simulink model "Straight_cs_old"  (R2016a)
settings: Solver=ode5  SolverMode=SingleTasking  StartTime=0.0  StopTime=30  FixedStep=1/1000  RelTol=1e-3
PreLoadFcn:
  | mbxruntime.callbacks.PreLoadFcn(bdroot);
PostLoadFcn:
  | mbxruntime.callbacks.PostLoadFcn(bdroot);
InitFcn:
  | mbxruntime.callbacks.InitFcn(bdroot);
StartFcn:
  | mbxruntime.callbacks.StartFcn(bdroot);
StopFcn:
  | mbxruntime.callbacks.StopFcn(bdroot);
model workspace (MAT data in the model file):
  mbox_table : struct (value not decoded)
  model_closed = 0
  sim_status = 0
values from neighbouring files (symbols this model uses):
  ACCDuration = 5    [PreScan_Runscript.m]
  V0 = ACCArray(2*ACCCasei-1)    [PreScan_Runscript.m]
  V1 = ACCArray(2*ACCCasei)    [PreScan_Runscript.m]
  VAccuracyIn = 0.8    [PreScan_Runscript.m]
  VDurationIn = 2    [PreScan_Runscript.m]
  VPIDIn = ACCArray(2*ACCCasei-1)    [PreScan_Runscript.m]
  VToleranceIn = 1    [PreScan_Runscript.m]
undefined symbols (not defined in the file or in its folder): ADASID, BMotor1, BMotor2, BrkDelayTime, DControlB, Delay1, Delay2, DiscIntNeverNeededParam, IControlB, JMotor1, JMotor2, mbxruntime, PControlB, PreScanCarSimLoadFcn, ratioGearF, ratioGearR, tabledata, TorqDelayTime, Tstep
undefined symbols (not defined in the file): SteeringColumn, SteeringWheel, WheelL0, WheelL1, WheelR0, WheelR1
libraries: simulink x14, simulink_extras x10, MyLib x3, PreScanSimulinkLibrary x3, Solver_SF x2, PreScanUsefulBlocks x2, pil_lib x1
(part 2 of 11)

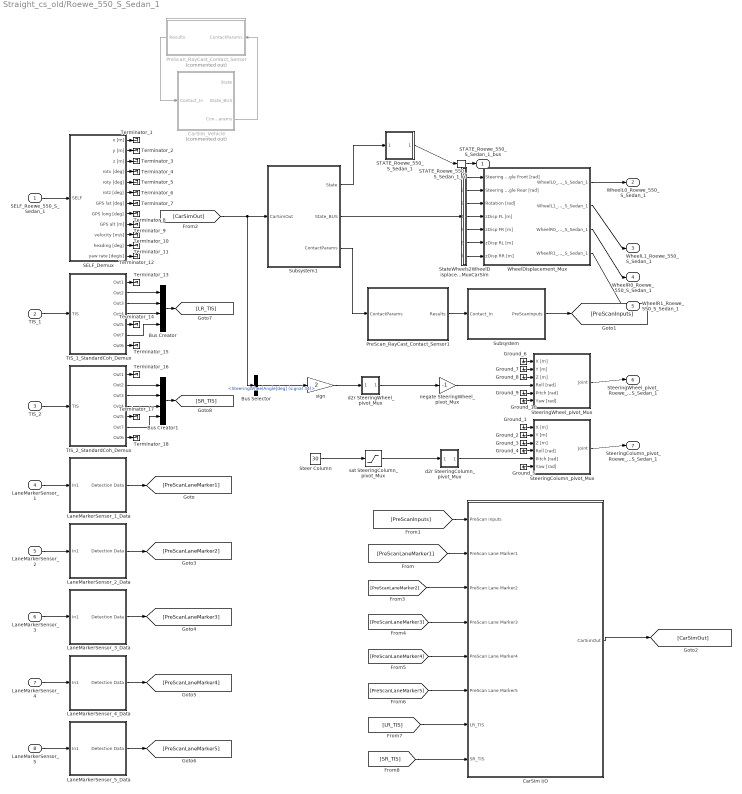
== system Straight_cs_old/Roewe_550_S_Sedan_1 ==
  SELF_Roewe_550_S_Sedan_1 : Inport  Tag=inport/SelfPort  OutDataTypeStr=Bus: PRESCAN_SELFSENSORDATA  PortDimensions=1  SampleTime=10/1000  BusOutputAsStruct=on
  TIS_1 : Inport  Tag=inport/TIS  Port=2  OutDataTypeStr=Bus: PRESCAN_SCANNERSENSOR_MESSAGE  PortDimensions=32  SampleTime=1/20  BusOutputAsStruct=on
  TIS_2 : Inport  Tag=inport/TIS  Port=3  OutDataTypeStr=Bus: PRESCAN_SCANNERSENSOR_MESSAGE  PortDimensions=32  SampleTime=1/20  BusOutputAsStruct=on
  LaneMarkerSensor_1 : Inport  Tag=inport/LaneMarker  Port=4  OutDataTypeStr=Bus: PRESCAN_LANEMARKER_MESSAGE  PortDimensions=4  SampleTime=1/20  BusOutputAsStruct=on
  LaneMarkerSensor_2 : Inport  Tag=inport/LaneMarker  Port=5  OutDataTypeStr=Bus: PRESCAN_LANEMARKER_MESSAGE  PortDimensions=4  SampleTime=1/20  BusOutputAsStruct=on
  LaneMarkerSensor_3 : Inport  Tag=inport/LaneMarker  Port=6  OutDataTypeStr=Bus: PRESCAN_LANEMARKER_MESSAGE  PortDimensions=4  SampleTime=1/20  BusOutputAsStruct=on
  LaneMarkerSensor_4 : Inport  Tag=inport/LaneMarker  Port=7  OutDataTypeStr=Bus: PRESCAN_LANEMARKER_MESSAGE  PortDimensions=4  SampleTime=1/20  BusOutputAsStruct=on
  LaneMarkerSensor_5 : Inport  Tag=inport/LaneMarker  Port=8  OutDataTypeStr=Bus: PRESCAN_LANEMARKER_MESSAGE  PortDimensions=4  SampleTime=1/20  BusOutputAsStruct=on
  Bus Creator : BusCreator  Inputs=4
  Bus Creator1 : BusCreator  Inputs=4
  Bus Selector : BusSelector  OutputSignals=SteeringWheelAngle[deg] (signal 34)
  CarSim I/O : Subsystem
  CarSim_Vehicle : Subsystem  Tag=UserSpecified_Subsys  Description=..\..\..\Program Files (x86)\CarSim201601_Data\Extensions\Simulink\CarSim_VehicleDynamics.mdl  Commented=on  LoadFcn=PreScanCarSimLoadFcn();  mask(User specified subsystem){update=off, sourcefilename=..\..\..\Program Files (x86)\CarSim201601_Data\Extensions\Simulink\CarSim_VehicleDynamics.mdl}
      mask prompts: update "Update (default: not checked)"; sourcefilename "Source file name"
      mask help:
      | A User-specified model may be selected as Controller or Dynamics of the vehicle. PreScan will copy the contents of the User-specified model into the user-specified model block.
      |
      | If update checkbox is checked the current user-specified model block will be deleted and will be REPLACED by (new) user specified model blocks. So, the current user specified model elements will be lost.
      |
      | Warning: If a new user-specified model is selected in the GUI, the user-specified model will be replaced.
      settings: DeleteFcn=PreScanBlockDeleteFcn;
      mask Help: eval('openHelp(227)')
      mask Display: userSpecifiedDynamics_mask_display();
  Ground_{1..10} (10 alike) : Ground
  LaneMarkerSensor_1_Data : Subsystem  Tag=demux/LaneMarkerSensor  mask{NUMBEROFSLICES=4, TimeStep=1/20}
      mask prompts: NUMBEROFSLICES "Number of slices"; TimeStep "Auto Assigned: Time Step [s]"
      mask Help: eval('openHelp(2301)')
  LaneMarkerSensor_2_Data : Subsystem  Tag=demux/LaneMarkerSensor  mask{NUMBEROFSLICES=4, TimeStep=1/20}
      mask prompts: NUMBEROFSLICES "Number of slices"; TimeStep "Auto Assigned: Time Step [s]"
      mask Help: eval('openHelp(2301)')
  LaneMarkerSensor_3_Data : Subsystem  Tag=demux/LaneMarkerSensor  mask{NUMBEROFSLICES=4, TimeStep=1/20}
      mask prompts: NUMBEROFSLICES "Number of slices"; TimeStep "Auto Assigned: Time Step [s]"
      mask Help: eval('openHelp(2301)')
  LaneMarkerSensor_4_Data : Subsystem  Tag=demux/LaneMarkerSensor  mask{NUMBEROFSLICES=4, TimeStep=1/20}
      mask prompts: NUMBEROFSLICES "Number of slices"; TimeStep "Auto Assigned: Time Step [s]"
      mask Help: eval('openHelp(2301)')
  LaneMarkerSensor_5_Data : Subsystem  Tag=demux/LaneMarkerSensor  mask{NUMBEROFSLICES=4, TimeStep=1/20}
      mask prompts: NUMBEROFSLICES "Number of slices"; TimeStep "Auto Assigned: Time Step [s]"
      mask Help: eval('openHelp(2301)')
  PreScan_RayCast_Contact_Sensor : Subsystem  Tag=PreScan_RayCast_Contact_Sensor  Commented=on  LoadFcn=|  mask(PreScan Block: PreScan RayCast Contact Sensor){x0=-95.5472, y0=-0.064154, z0=0, Roll0=0, Pitch0=0, Yaw0=0, wheelRadius=0.44999998807907104, hcog=0, b=2.7049999237060547, TimeStep=-1}
      | load PrescanXYZData;
      | load PrescanRPYData;
      | load PrescanQuatData;
      | load PrescanAxisAngleData;
      | load PrescanPoseData;
      | load PrescanPoseQData;
      | load PrescanPoseAData;
      | load PrescanWheelContactData;
      mask prompts: x0 "Ini x-position VEHICLE wrt GLOBAL axis system [m]"; y0 "Ini y-position VEHICLE wrt GLOBAL axis system [m]"; z0 "Ini z-position VEHICLE wrt GLOBAL axis system [m]"; Roll0 "Ini roll-angle BODY wrt VEHICLE axis system [deg]"; Pitch0 "Ini pitch-angle BODY wrt VEHICLE axis system [deg]"; Yaw0 "Ini yaw-angle VEHICLE wrt GLOBAL axis system [deg]"; wheelRadius "Wheel Radius [m]"; hcog "Dynamics: hCoG [m]"; b "Dynamics: b [m]"; TimeStep "Time Step [s]"
      mask help:
      | This block encapsulates the base Contact sensor.
      |
      | It takes input parameters from the PreScan 3D vehicle dynamics block and outputs contact results.
      mask Help: eval('openHelp(251)')
  PreScan_RayCast_Contact_Sensor1 : Subsystem  Tag=PreScan_RayCast_Contact_Sensor  LoadFcn=|  mask(PreScan Block: PreScan RayCast Contact Sensor){x0=-2.6473, y0=0.062788, z0=0, Roll0=0, Pitch0=0, Yaw0=0, wheelRadius=0.44999998807907104, hcog=0, b=2.7049999237060547, TimeStep=-1}
      | load PrescanXYZData;
      | load PrescanRPYData;
      | load PrescanQuatData;
      | load PrescanAxisAngleData;
      | load PrescanPoseData;
      | load PrescanPoseQData;
      | load PrescanPoseAData;
      | load PrescanWheelContactData;
      mask prompts: x0 "Ini x-position VEHICLE wrt GLOBAL axis system [m]"; y0 "Ini y-position VEHICLE wrt GLOBAL axis system [m]"; z0 "Ini z-position VEHICLE wrt GLOBAL axis system [m]"; Roll0 "Ini roll-angle BODY wrt VEHICLE axis system [deg]"; Pitch0 "Ini pitch-angle BODY wrt VEHICLE axis system [deg]"; Yaw0 "Ini yaw-angle VEHICLE wrt GLOBAL axis system [deg]"; wheelRadius "Wheel Radius [m]"; hcog "Dynamics: hCoG [m]"; b "Dynamics: b [m]"; TimeStep "Time Step [s]"
      mask help:
      | This block encapsulates the base Contact sensor.
      |
      | It takes input parameters from the PreScan 3D vehicle dynamics block and outputs contact results.
      mask Help: eval('openHelp(251)')
  SELF_Demux : Subsystem  Tag=demux/SelfPort  mask(PreScan Demux Block:){}
      mask help:
      | The SELF port shows (state) information of the actor itself. The outputs are position in the experiment's axis system and the GPS coordinates, and the object's absolute velocity and compass heading.
      |
      | For more information, please click Help.
      settings: DeleteFcn=PreScanBlockDeleteFcn;
      mask Help: eval('openHelp(462)')
      mask Display:
      | port_label('output',1,'x [m]')
      | port_label('output',2,'y [m]')
      | port_label('output',3,'z [m]','texmode','on')
      | port_label('output',4,'Rotx [deg]','texmode','on')
      | port_label('output',5,'Roty [deg]','texmode','on')
      | port_label('output',6,'Rotz [deg]','texmode','on')
      | port_label('output',7,'GPS lat [deg]','texmode','on')
      | port_label('output',8,'GPS long [deg]','texmode','on')
      | port_label('output',9,'GPS alt [m]','texmode','on')
      | port_label('output',10,'Velocity [m/s]')
      | port_label('output',11,'Heading [deg]')
      | port_label('output',12,'Yaw rate [deg/s]')
  STATE_Roewe_550_S_Sedan_1 : Subsystem  Tag=mux/StatePort  Priority=0  LoadFcn=load PrescanStateActuatorData  mask(PreScan Sink Block: State){x0=-95.5472, y0=-0.064154, z0=0, Roll0=0, Pitch0=0, Yaw0=0, TimeStep=1/1000}
      mask prompts: x0 "Ini x-position VEHICLE wrt GLOBAL axis system [m]"; y0 "Ini y-position VEHICLE wrt GLOBAL axis system [m]"; z0 "Ini z-position VEHICLE wrt GLOBAL axis system [m]"; Roll0 "Ini roll-angle BODY wrt VEHICLE axis system [deg]"; Pitch0 "Ini pitch-angle BODY wrt VEHICLE axis system [deg]"; Yaw0 "Ini yaw-angle VEHICLE wrt GLOBAL axis system [deg]"; TimeStep "Auto-Assigned: Upload Period [s]"
      mask help:
      | The Actor State contains a vector signal of size (9x1), containing the following signals:
      |
      | -  Position                  (x,y,z)                                     [m]
      | -  Velocity                  (vx,vy,vz)                               [m/s]
      | -  Angles                    (Roll, Pitch, Yaw)                   [rad]
      |
      | The Actor state is defined in the global axis system.
      | The state is superponed on the Initial position defined in the GUI.
      |
      | For more information, please click Help.
      settings: DeleteFcn=PreScanBlockDeleteFcn;
      mask Help: eval('openHelp(222)')
      mask Display: image(imread('State.png'))
  STATE_Roewe_550_S_Sedan_1_rc : RateTransition  Tag=mux_rc/StatePort  OutPortSampleTimeOpt=Inherit
  StateWheels2WheelDisplacementMuxCarSim : Subsystem  Tag=StateWheels2WheelDisplacementMuxCarSim  mask(PreScan Utility Block:){}
      mask help: This block selects the CarSim wheels displacement and rotation.
      settings: DeleteFcn=PreScanBlockDeleteFcn;
  Steer Column : Constant  Value=30
  SteeringColumn_pivot_Mux : Subsystem  Tag=mux/Joint  mask(PreScan Mux Block){DisplayName=SteeringColumn}
      mask prompts: DisplayName "Display Name"
      mask help:
      | This block simulates a generic joint used for generic models. This joint can be enabled/disabled from the GUI.
      |
      | For more information, please click Help.
      settings: DeleteFcn=PreScanBlockDeleteFcn;
      mask Help: eval('openHelp(254)')
  SteeringWheel_pivot_Mux : Subsystem  Tag=mux/Joint  mask(PreScan Mux Block){DisplayName=SteeringWheel}
      mask prompts: DisplayName "Display Name"
      mask help:
      | This block simulates a generic joint used for generic models. This joint can be enabled/disabled from the GUI.
      |
      | For more information, please click Help.
      settings: DeleteFcn=PreScanBlockDeleteFcn;
      mask Help: eval('openHelp(254)')
  Subsystem : Subsystem
  Subsystem1 : Subsystem
  TIS_1_StandardCoh_Demux : Subsystem  Tag=demux/TIS/StandardCoh  TreatAsAtomicUnit=on  mask(PreScan Demux Block: TIS){MAXMESSAGES=32}
      mask prompts: MAXMESSAGES "Number of Objects"
      mask Help: eval('openHelp(449)')
      mask Display:
      | port_label('input',1,'TIS')
      | port_label('output',1,'Beam ID [-]')
      | port_label('output',2,'Range [m]')
      | port_label('output',3,'DopplerVelocity [m/s]')
      | port_label('output',4,'{\theta} [deg]','texmode','on')
      | port_label('output',5,'{\phi} [deg]','texmode','on')
      | port_label('output',6,'Target ID [-]','texmode','on')
      | port_label('output',7,'TIS Data','texmode','on')
  TIS_2_StandardCoh_Demux : Subsystem  Tag=demux/TIS/StandardCoh  TreatAsAtomicUnit=on  mask(PreScan Demux Block: TIS){MAXMESSAGES=32}
      mask prompts: MAXMESSAGES "Number of Objects"
      mask Help: eval('openHelp(449)')
      mask Display:
      | port_label('input',1,'TIS')
      | port_label('output',1,'Beam ID [-]')
      | port_label('output',2,'Range [m]')
      | port_label('output',3,'DopplerVelocity [m/s]')
      | port_label('output',4,'{\theta} [deg]','texmode','on')
      | port_label('output',5,'{\phi} [deg]','texmode','on')
      | port_label('output',6,'Target ID [-]','texmode','on')
      | port_label('output',7,'TIS Data','texmode','on')
  Terminator_{1..18} (18 alike) : Terminator
  WheelDisplacement_Mux : Subsystem  Tag=mux/JointGroup  mask(JointGroup){}
      mask help:
      | The JointGroup allows to control several Joints in one go, as defined for this particular model.
      | For more information, look in the PreScan manual in the section "Model Preparation Tool" -> "Joint Groups"
      |
      | For more information on the Joints simulink interface, press Help.
      mask Help: eval('openHelp(254)')
  d2r SteeringColumn_pivot_Mux : Subsystem  mask(DegreesToRadians){}
      mask help: SimulinkBlocks:simulink_extras:DegreesToRadians_MD
      mask Help: web([docroot '/simulink/ref_extras/degreestoradians.html'])
      mask Display: disp('D2R')
  d2r SteeringWheel_pivot_Mux : Subsystem  mask(DegreesToRadians){}
      mask help: SimulinkBlocks:simulink_extras:DegreesToRadians_MD
      mask Help: web([docroot '/simulink/ref_extras/degreestoradians.html'])
      mask Display: disp('D2R')
  negate SteeringWheel_pivot_Mux : Gain  Gain=-1
  sat SteeringColumn_pivot_Mux : Saturate  UpperLimit=30  LowerLimit=-5
  sign : Gain  Gain=2
  STATE_Roewe_550_S_Sedan_1_bus : Outport  Tag=outport/StatePort  OutDataTypeStr=Bus: PRESCAN_STATEACTUATORDATA  PortDimensions=1  SampleTime=10/1000
  WheelL0_Roewe_550_S_Sedan_1 : Outport  Tag=outport/JointActuator  Port=2  OutDataTypeStr=Bus: PRESCAN_POSE_DATA  SampleTime=10/1000
  WheelL1_Roewe_550_S_Sedan_1 : Outport  Tag=outport/JointActuator  Port=3  OutDataTypeStr=Bus: PRESCAN_POSE_DATA  SampleTime=10/1000
  WheelR0_Roewe_550_S_Sedan_1 : Outport  Tag=outport/JointActuator  Port=4  OutDataTypeStr=Bus: PRESCAN_POSE_DATA  SampleTime=10/1000
  WheelR1_Roewe_550_S_Sedan_1 : Outport  Tag=outport/JointActuator  Port=5  OutDataTypeStr=Bus: PRESCAN_POSE_DATA  SampleTime=10/1000
  SteeringWheel_pivot_Roewe_550_S_Sedan_1 : Outport  Tag=outport/JointActuator  Port=6  OutDataTypeStr=Bus: PRESCAN_POSE_DATA  SampleTime=10/1000
  SteeringColumn_pivot_Roewe_550_S_Sedan_1 : Outport  Tag=outport/JointActuator  Port=7  OutDataTypeStr=Bus: PRESCAN_POSE_DATA  SampleTime=10/1000
  wires:
  LaneMarkerSensor_1_Data/1(Detection Data) -> [PreScanLaneMarker1]
  LaneMarkerSensor_2_Data/1(Detection Data) -> [PreScanLaneMarker2]
  LaneMarkerSensor_3_Data/1(Detection Data) -> [PreScanLaneMarker3]
  LaneMarkerSensor_4_Data/1(Detection Data) -> [PreScanLaneMarker4]
  LaneMarkerSensor_5_Data/1(Detection Data) -> [PreScanLaneMarker5]
  [PreScanLaneMarker1] -> CarSim I/O/2(PreScan Lane Marker1)
  [PreScanInputs] -> CarSim I/O/1(PreScan inputs)
  Subsystem/1(PreScanInputs) -> [PreScanInputs]
  [CarSimOut] -> Subsystem1/1(CarSimOut), Bus Selector/1
  PreScan_RayCast_Contact_Sensor1/1(Results) -> Subsystem/1(Contact_In)
  Subsystem1/3(ContactParams) -> PreScan_RayCast_Contact_Sensor1/1(ContactParams)
  Subsystem1/1(State) -> STATE_Roewe_550_S_Sedan_1/1(State)
  Subsystem1/2(State_BUS) -> StateWheels2WheelDisplacementMuxCarSim/1(StateWheels)
  CarSim I/O/1(CarSimOut) -> [CarSimOut]
  [PreScanLaneMarker2] -> CarSim I/O/3(PreScan Lane Marker2)
  [PreScanLaneMarker3] -> CarSim I/O/4(PreScan Lane Marker3)
  [PreScanLaneMarker4] -> CarSim I/O/5(PreScan Lane Marker4)
  [PreScanLaneMarker5] -> CarSim I/O/6(PreScan Lane Marker5)
  TIS_1_StandardCoh_Demux/2(Out2) -> Bus Creator/1
  TIS_1_StandardCoh_Demux/3(Out3) -> Bus Creator/2
  TIS_1_StandardCoh_Demux/4(Out4) -> Bus Creator/3
  TIS_1_StandardCoh_Demux/6(Out7) -> Bus Creator/4
  TIS_2_StandardCoh_Demux/2(Out2) -> Bus Creator1/1
  TIS_2_StandardCoh_Demux/3(Out3) -> Bus Creator1/2
  TIS_2_StandardCoh_Demux/4(Out4) -> Bus Creator1/3
  TIS_2_StandardCoh_Demux/6(Out7) -> Bus Creator1/4
  negate SteeringWheel_pivot_Mux/1 -> SteeringWheel_pivot_Mux/4(Roll [rad])
  d2r SteeringWheel_pivot_Mux/1(Radians out) -> negate SteeringWheel_pivot_Mux/1
  Bus Selector/1 -> sign/1  "<SteeringWheelAngle[deg] (signal 34)>"
  sign/1 -> d2r SteeringWheel_pivot_Mux/1(Degrees in)
  d2r SteeringColumn_pivot_Mux/1(Radians out) -> SteeringColumn_pivot_Mux/5(Pitch [rad])
  sat SteeringColumn_pivot_Mux/1 -> d2r SteeringColumn_pivot_Mux/1(Degrees in)
  Steer Column/1 -> sat SteeringColumn_pivot_Mux/1
  Bus Creator/1 -> [LR_TIS]
  Bus Creator1/1 -> [SR_TIS]
  [LR_TIS] -> CarSim I/O/7(LR_TIS)
  [SR_TIS] -> CarSim I/O/8(SR_TIS)
  STATE_Roewe_550_S_Sedan_1_rc/1 -> STATE_Roewe_550_S_Sedan_1_bus/1
  STATE_Roewe_550_S_Sedan_1/1(StateBus) -> STATE_Roewe_550_S_Sedan_1_rc/1
  SELF_Roewe_550_S_Sedan_1/1 -> SELF_Demux/1(SELF)
  TIS_1/1 -> TIS_1_StandardCoh_Demux/1(TIS)
  TIS_2/1 -> TIS_2_StandardCoh_Demux/1(TIS)
  LaneMarkerSensor_1/1 -> LaneMarkerSensor_1_Data/1(In1)
  LaneMarkerSensor_2/1 -> LaneMarkerSensor_2_Data/1(In1)
  LaneMarkerSensor_3/1 -> LaneMarkerSensor_3_Data/1(In1)
  LaneMarkerSensor_4/1 -> LaneMarkerSensor_4_Data/1(In1)
  LaneMarkerSensor_5/1 -> LaneMarkerSensor_5_Data/1(In1)
  WheelDisplacement_Mux/1(WheelL0_Roewe_550_S_Sedan_1) -> WheelL0_Roewe_550_S_Sedan_1/1
  WheelDisplacement_Mux/2(WheelL1_Roewe_550_S_Sedan_1) -> WheelL1_Roewe_550_S_Sedan_1/1
  WheelDisplacement_Mux/3(WheelR0_Roewe_550_S_Sedan_1) -> WheelR0_Roewe_550_S_Sedan_1/1
  WheelDisplacement_Mux/4(WheelR1_Roewe_550_S_Sedan_1) -> WheelR1_Roewe_550_S_Sedan_1/1
  SteeringWheel_pivot_Mux/1(Joint) -> SteeringWheel_pivot_Roewe_550_S_Sedan_1/1
  SteeringColumn_pivot_Mux/1(Joint) -> SteeringColumn_pivot_Roewe_550_S_Sedan_1/1
  CarSim_Vehicle/3(ContactParams) -> PreScan_RayCast_Contact_Sensor/1(ContactParams)
  PreScan_RayCast_Contact_Sensor/1(Results) -> CarSim_Vehicle/1(Contact_In)
  StateWheels2WheelDisplacementMuxCarSim/1(Steering_Angle_Front_[rad]) -> WheelDisplacement_Mux/1(Steering Angle Front [rad])
  StateWheels2WheelDisplacementMuxCarSim/2(Steering_Angle_Rear_[rad]) -> WheelDisplacement_Mux/2(Steering Angle Rear [rad])
  StateWheels2WheelDisplacementMuxCarSim/3(WheelsRotation_[rad]) -> WheelDisplacement_Mux/3(Rotation [rad])
  StateWheels2WheelDisplacementMuxCarSim/4(z displacement FL [m]) -> WheelDisplacement_Mux/4(zDisp FL [m])
  StateWheels2WheelDisplacementMuxCarSim/5(z displacement FR [m]) -> WheelDisplacement_Mux/5(zDisp FR [m])
  StateWheels2WheelDisplacementMuxCarSim/6(z displacement RL [m]) -> WheelDisplacement_Mux/6(zDisp RL [m])
  StateWheels2WheelDisplacementMuxCarSim/7(z displacement RR [m]) -> WheelDisplacement_Mux/7(zDisp RR [m])
  SELF_Demux/1(x [m]) -> Terminator_1/1
  SELF_Demux/2(y [m]) -> Terminator_2/1
  SELF_Demux/3(z [m]) -> Terminator_3/1
  SELF_Demux/4(rotx [deg]) -> Terminator_4/1
  SELF_Demux/5(roty [deg]) -> Terminator_5/1
  SELF_Demux/6(rotz [deg]) -> Terminator_6/1
  SELF_Demux/7(GPS lat [deg]) -> Terminator_7/1
  SELF_Demux/8(GPS long [deg]) -> Terminator_8/1
  SELF_Demux/9(GPS alt [m]) -> Terminator_9/1
  SELF_Demux/10(velocity [m/s]) -> Terminator_10/1
  SELF_Demux/11(heading [deg]) -> Terminator_11/1
  SELF_Demux/12(yaw rate [deg/s]) -> Terminator_12/1
  Ground_1/1 -> SteeringColumn_pivot_Mux/1(X [m])
  Ground_2/1 -> SteeringColumn_pivot_Mux/2(Y [m])
  Ground_3/1 -> SteeringColumn_pivot_Mux/3(Z [m])
  Ground_4/1 -> SteeringColumn_pivot_Mux/4(Roll [rad])
  Ground_5/1 -> SteeringColumn_pivot_Mux/6(Yaw [rad])
  Ground_6/1 -> SteeringWheel_pivot_Mux/1(X [m])
  Ground_7/1 -> SteeringWheel_pivot_Mux/2(Y [m])
  Ground_8/1 -> SteeringWheel_pivot_Mux/3(Z [m])
  Ground_9/1 -> SteeringWheel_pivot_Mux/5(Pitch [rad])
  Ground_10/1 -> SteeringWheel_pivot_Mux/6(Yaw [rad])
  TIS_1_StandardCoh_Demux/1(Out1) -> Terminator_13/1
  TIS_1_StandardCoh_Demux/5(Out5) -> Terminator_14/1
  TIS_1_StandardCoh_Demux/7(Out6) -> Terminator_15/1
  TIS_2_StandardCoh_Demux/1(Out1) -> Terminator_16/1
  TIS_2_StandardCoh_Demux/5(Out5) -> Terminator_17/1
  TIS_2_StandardCoh_Demux/7(Out6) -> Terminator_18/1

== system Straight_cs_old/SELF_Roewe_550_S_Sedan_1 ==
  Sensor : S-Function  FunctionName=sfun_SelfSensor  Parameters=UniqueID, TimeStep  SFunctionDeploymentMode=off  EnableBusSupport=off  mask(PreScan Source Block: SELF){UniqueID=29, TimeStep=10/1000}
      mask prompts: UniqueID "Auto-Assigned: Unique ID"; TimeStep "Auto-Assigned: Upload Period [s]"
      mask help:
      | The SELF port shows (state) information of the actor itself. The outputs are position in the experiment's axis system and the GPS coordinates, and the object's absolute velocity and compass heading.
      |
      | For more information, please click Help.
      mask Help: eval('openHelp(462)')
      mask Display: image(imread('GPS.png'))
  SELF_Roewe_550_S_Sedan_1 : Outport  Tag=outport/SelfPort  OutDataTypeStr=Bus: PRESCAN_SELFSENSORDATA  PortDimensions=1  SampleTime=10/1000
  wires:
  Sensor/1 -> SELF_Roewe_550_S_Sedan_1/1

== system Straight_cs_old/STATE_Roewe_550_S_Sedan_1_bus ==
  STATE_Roewe_550_S_Sedan_1_bus : Inport  Tag=inport/StatePort  OutDataTypeStr=Bus: PRESCAN_STATEACTUATORDATA  PortDimensions=1  SampleTime=10/1000  BusOutputAsStruct=on
  Actuator : S-Function  FunctionName=sfun_StateActuator  Parameters=UniqueID, TimeStep  SFunctionDeploymentMode=off  EnableBusSupport=off  mask(PreScan Sink Block: State){UniqueID=29, TimeStep=10/1000}
      mask prompts: UniqueID "Auto-Assigned: Unique ID"; TimeStep "Auto-Assigned: Upload Period [s]"
      mask help:
      | The Actor State contains a vector signal of size (9x1), containing the following signals:
      |
      | -  Position    	(x,y,z)             	[m]
      | -  Velocity    	(vx,vy,vz)         	[m/s]
      | -  Angles       	(Roll, Pitch, Yaw)	[rad]
      |
      | The Actor state is defined in the global axis system.
      | The state is superponed on the Initial position defined in the GUI.
      |
      | For more information, please click Help.
      mask Help: eval('openHelp(222)')
      mask Display: image(imread('State.png'))
  wires:
  STATE_Roewe_550_S_Sedan_1_bus/1 -> Actuator/1

== system Straight_cs_old/SteeringColumn_pivot_Roewe_550_S_Sedan_1 ==
  SteeringColumn_pivot_Roewe_550_S_Sedan_1 : Inport  Tag=inport/JointActuator  OutDataTypeStr=Bus: PRESCAN_POSE_DATA  SampleTime=10/1000  BusOutputAsStruct=on
  Actuator : Subsystem  Tag=VisuJoint  mask(PreScan Sink Block: VisuJoint){UniqueID=29, Translate_ObjectID3D=Roewe_550_S_Sedan_1.SteeringColumn_pivot, Rotate_ObjectID3D=Roewe_550_S_Sedan_1.SteeringColumn_pivot, TimeStep=10/1000, DisplayName=[]}
      mask prompts: UniqueID "Parent Unique ID"; Translate_ObjectID3D "Translate Object Name"; Rotate_ObjectID3D "Rotate Object Name"; TimeStep "Simulation Step"; DisplayName "Display Name"
      mask help:
      | The VisuJoint block provides a way to adapt the location and orientation of a part of an object.
      |
      | For more information, please click Help.
      settings: DeleteFcn=PreScanBlockDeleteFcn;
      mask Help: eval('openHelp(223)')
      mask Display: image(imread('Joint.png'))
  wires:
  SteeringColumn_pivot_Roewe_550_S_Sedan_1/1 -> Actuator/1(Joint)

== system Straight_cs_old/SteeringWheel_pivot_Roewe_550_S_Sedan_1 ==
  SteeringWheel_pivot_Roewe_550_S_Sedan_1 : Inport  Tag=inport/JointActuator  OutDataTypeStr=Bus: PRESCAN_POSE_DATA  SampleTime=10/1000  BusOutputAsStruct=on
  Actuator : Subsystem  Tag=VisuJoint  mask(PreScan Sink Block: VisuJoint){UniqueID=29, Translate_ObjectID3D=Roewe_550_S_Sedan_1.SteeringWheel_pivot, Rotate_ObjectID3D=Roewe_550_S_Sedan_1.SteeringWheel_pivot, TimeStep=10/1000, DisplayName=[]}
      mask prompts: UniqueID "Parent Unique ID"; Translate_ObjectID3D "Translate Object Name"; Rotate_ObjectID3D "Rotate Object Name"; TimeStep "Simulation Step"; DisplayName "Display Name"
      mask help:
      | The VisuJoint block provides a way to adapt the location and orientation of a part of an object.
      |
      | For more information, please click Help.
      settings: DeleteFcn=PreScanBlockDeleteFcn;
      mask Help: eval('openHelp(223)')
      mask Display: image(imread('Joint.png'))
  wires:
  SteeringWheel_pivot_Roewe_550_S_Sedan_1/1 -> Actuator/1(Joint)

== system Straight_cs_old/Synchronizer ==
  Bus Selector1 : BusSelector  OutputSignals=FederateStopped
  Stop Simulation : Stop
  sfun_Synchronizer : S-Function  FunctionName=sfun_Synchronizer  Parameters=SampleTime  SFunctionDeploymentMode=off  EnableBusSupport=off  mask(Legacy Function){SFunctionSpec=void prescan_synchronizer_outputFcn(void ** work1, PRESCAN_SYNCHRONIZEDATA y1[1]), SampleTime=TimeStep, ShowSpec=on}
      mask prompts: SampleTime "Sample time (-1 for inherited):"; ShowSpec "Display function specification"
      mask help:
      | This block allows you to call the legacy functions specified by the following Legacy Code Tool definition:
      | def.SFunctionName = 'sfun_Synchronizer';
      | def.OutputFcnSpec = 'void prescan_synchronizer_outputFcn(void ** work1, PRESCAN_SYNCHRONIZEDATA y1[1])';
      | def.StartFcnSpec = 'void prescan_synchronizer_startFcn(void ** work1)';
      | def.TerminateFcnSpec = 'void prescan_synchronizer_terminateFcn(void ** work1)';
      | def.HeaderFiles = {'prescan_synchronizer_data.h'};
      | def.HostLibFiles = {'sensorinterfaced.lib'};
      | def.IncPaths = {'src', 'C:\prescandev\vislibrary\vis\..\pimp\include\sensors\InterfaceRTW'};
      | def.SrcPaths = {'src'};
      | def.LibPaths = {'C:\\prescandev\\vislibrary_build\lib'};
      | def.SampleTime = 'parameterized';
      | def.Options.language = 'C';
      mask Help: <p>This block was generated automatically by the Legacy Code Tool. For detailed help on this tool, call<a href="matlab:legacy_code('help')"> legacy_code('help')</a>.</p>
      mask Callback ShowSpec:
      | if strcmp(get_param(gcbh, 'ShowSpec'), 'on')
      |   set_param(gcbh, 'MaskDisplay', sprintf('fprintf(''%s'');', get_param(gcbh, 'SFunctionSpec')));
      | else
      |   set_param(gcbh, 'MaskDisplay', sprintf('fprintf(''%s'');', get_param(gcbh, 'FunctionName')));
      | end
      mask Display: fprintf('void prescan_synchronizer_outputFcn(void ** work1, PRESCAN_SYNCHRONIZEDATA y1[1])');
  wires:
  Bus Selector1/1 -> Stop Simulation/1  "<FederateStopped>"
  sfun_Synchronizer/1 -> Bus Selector1/1

== system Straight_cs_old/TIS_1 ==
  Sensor : S-Function  FunctionName=sfun_TIS  Parameters=sensorID, detectableObjects, timestep  SFunctionDeploymentMode=off  EnableBusSupport=off  mask(PreScan Source Block: Technology Independent Sensor (TIS)){sensorID=1876, detectableObjects=32, timestep=1/20}
      mask prompts: sensorID "Sensor ID"; detectableObjects "Max detectable objects:"; timestep "MATLAB timestep:"
      mask help:
      | The Technology Independent Sensor (TIS) provides a sensor with all sensor-related influence factors (like noise, drift and accuracy) without being technology specific (like radar and lidar). The TIS detects the closest point on the geometry of an object.
      |
      | For more information, please click Help.
      mask Help: eval('openHelp(449)')
      mask Display: image(imread('TIS.png'))
  TIS_1 : Outport  Tag=outport/TIS  OutDataTypeStr=Bus: PRESCAN_SCANNERSENSOR_MESSAGE  PortDimensions=32  SampleTime=1/20
  wires:
  Sensor/1 -> TIS_1/1

== system Straight_cs_old/TIS_2 ==
  Sensor : S-Function  FunctionName=sfun_TIS  Parameters=sensorID, detectableObjects, timestep  SFunctionDeploymentMode=off  EnableBusSupport=off  mask(PreScan Source Block: Technology Independent Sensor (TIS)){sensorID=1877, detectableObjects=32, timestep=1/20}
      mask prompts: sensorID "Sensor ID"; detectableObjects "Max detectable objects:"; timestep "MATLAB timestep:"
      mask help:
      | The Technology Independent Sensor (TIS) provides a sensor with all sensor-related influence factors (like noise, drift and accuracy) without being technology specific (like radar and lidar). The TIS detects the closest point on the geometry of an object.
      |
      | For more information, please click Help.
      mask Help: eval('openHelp(449)')
      mask Display: image(imread('TIS.png'))
  TIS_2 : Outport  Tag=outport/TIS  OutDataTypeStr=Bus: PRESCAN_SCANNERSENSOR_MESSAGE  PortDimensions=32  SampleTime=1/20
  wires:
  Sensor/1 -> TIS_2/1

== system Straight_cs_old/TrafficLightDoubleUS_1 ==
  Ground_{1..6} (6 alike) : Ground
  VISUCasingLights_1_Mux : Subsystem  Tag=mux/VisuCasingLights  mask(PreScan User Interface: VisuTrafficLight){}
      mask help:
      | The VisuTrafficLight block provides a way to animate traffic lights: switch on and off individual lights.
      |
      | For more information, please click Help.
      mask Help: eval('openHelp(731)')
  VISUCasingLights_2_Mux : Subsystem  Tag=mux/VisuCasingLights  mask(PreScan User Interface: VisuTrafficLight){}
      mask help:
      | The VisuTrafficLight block provides a way to animate traffic lights: switch on and off individual lights.
      |
      | For more information, please click Help.
      mask Help: eval('openHelp(731)')
  VISUCasingLights_1_TrafficLightDoubleUS_1 : Outport  Tag=outport/VisuCasingLights  SampleTime=10/1000
  VISUCasingLights_2_TrafficLightDoubleUS_1 : Outport  Tag=outport/VisuCasingLights  Port=2  SampleTime=10/1000
  wires:
  VISUCasingLights_1_Mux/1(VISUCasingLights_1_TrafficLightDoubleUS_1) -> VISUCasingLights_1_TrafficLightDoubleUS_1/1
  VISUCasingLights_2_Mux/1(VISUCasingLights_2_TrafficLightDoubleUS_1) -> VISUCasingLights_2_TrafficLightDoubleUS_1/1
  Ground_1/1 -> VISUCasingLights_1_Mux/1(Green [-])
  Ground_2/1 -> VISUCasingLights_1_Mux/2(Orange [-])
  Ground_3/1 -> VISUCasingLights_1_Mux/3(Red [-])
  Ground_4/1 -> VISUCasingLights_2_Mux/1(Green [-])
  Ground_5/1 -> VISUCasingLights_2_Mux/2(Orange [-])
  Ground_6/1 -> VISUCasingLights_2_Mux/3(Red [-])

== system Straight_cs_old/TrafficLightDoubleUS_2 ==
  Ground_{1..6} (6 alike) : Ground
  VISUCasingLights_1_Mux : Subsystem  Tag=mux/VisuCasingLights  mask(PreScan User Interface: VisuTrafficLight){}
      mask help:
      | The VisuTrafficLight block provides a way to animate traffic lights: switch on and off individual lights.
      |
      | For more information, please click Help.
      mask Help: eval('openHelp(731)')
  VISUCasingLights_2_Mux : Subsystem  Tag=mux/VisuCasingLights  mask(PreScan User Interface: VisuTrafficLight){}
      mask help:
      | The VisuTrafficLight block provides a way to animate traffic lights: switch on and off individual lights.
      |
      | For more information, please click Help.
      mask Help: eval('openHelp(731)')
  VISUCasingLights_1_TrafficLightDoubleUS_2 : Outport  Tag=outport/VisuCasingLights  SampleTime=10/1000
  VISUCasingLights_2_TrafficLightDoubleUS_2 : Outport  Tag=outport/VisuCasingLights  Port=2  SampleTime=10/1000
  wires:
  VISUCasingLights_1_Mux/1(VISUCasingLights_1_TrafficLightDoubleUS_2) -> VISUCasingLights_1_TrafficLightDoubleUS_2/1
  VISUCasingLights_2_Mux/1(VISUCasingLights_2_TrafficLightDoubleUS_2) -> VISUCasingLights_2_TrafficLightDoubleUS_2/1
  Ground_1/1 -> VISUCasingLights_1_Mux/1(Green [-])
  Ground_2/1 -> VISUCasingLights_1_Mux/2(Orange [-])
  Ground_3/1 -> VISUCasingLights_1_Mux/3(Red [-])
  Ground_4/1 -> VISUCasingLights_2_Mux/1(Green [-])
  Ground_5/1 -> VISUCasingLights_2_Mux/2(Orange [-])
  Ground_6/1 -> VISUCasingLights_2_Mux/3(Red [-])

== system Straight_cs_old/TrafficLightDoubleUS_3 ==
  Ground_{1..6} (6 alike) : Ground
  VISUCasingLights_1_Mux : Subsystem  Tag=mux/VisuCasingLights  mask(PreScan User Interface: VisuTrafficLight){}
      mask help:
      | The VisuTrafficLight block provides a way to animate traffic lights: switch on and off individual lights.
      |
      | For more information, please click Help.
      mask Help: eval('openHelp(731)')
  VISUCasingLights_2_Mux : Subsystem  Tag=mux/VisuCasingLights  mask(PreScan User Interface: VisuTrafficLight){}
      mask help:
      | The VisuTrafficLight block provides a way to animate traffic lights: switch on and off individual lights.
      |
      | For more information, please click Help.
      mask Help: eval('openHelp(731)')
  VISUCasingLights_1_TrafficLightDoubleUS_3 : Outport  Tag=outport/VisuCasingLights  SampleTime=10/1000
  VISUCasingLights_2_TrafficLightDoubleUS_3 : Outport  Tag=outport/VisuCasingLights  Port=2  SampleTime=10/1000
  wires:
  VISUCasingLights_1_Mux/1(VISUCasingLights_1_TrafficLightDoubleUS_3) -> VISUCasingLights_1_TrafficLightDoubleUS_3/1
  VISUCasingLights_2_Mux/1(VISUCasingLights_2_TrafficLightDoubleUS_3) -> VISUCasingLights_2_TrafficLightDoubleUS_3/1
  Ground_1/1 -> VISUCasingLights_1_Mux/1(Green [-])
  Ground_2/1 -> VISUCasingLights_1_Mux/2(Orange [-])
  Ground_3/1 -> VISUCasingLights_1_Mux/3(Red [-])
  Ground_4/1 -> VISUCasingLights_2_Mux/1(Green [-])
  Ground_5/1 -> VISUCasingLights_2_Mux/2(Orange [-])
  Ground_6/1 -> VISUCasingLights_2_Mux/3(Red [-])

== system Straight_cs_old/TrafficLightDoubleUS_4 ==
  Ground_{1..6} (6 alike) : Ground
  VISUCasingLights_1_Mux : Subsystem  Tag=mux/VisuCasingLights  mask(PreScan User Interface: VisuTrafficLight){}
      mask help:
      | The VisuTrafficLight block provides a way to animate traffic lights: switch on and off individual lights.
      |
      | For more information, please click Help.
      mask Help: eval('openHelp(731)')
  VISUCasingLights_2_Mux : Subsystem  Tag=mux/VisuCasingLights  mask(PreScan User Interface: VisuTrafficLight){}
      mask help:
      | The VisuTrafficLight block provides a way to animate traffic lights: switch on and off individual lights.
      |
      | For more information, please click Help.
      mask Help: eval('openHelp(731)')
  VISUCasingLights_1_TrafficLightDoubleUS_4 : Outport  Tag=outport/VisuCasingLights  SampleTime=10/1000
  VISUCasingLights_2_TrafficLightDoubleUS_4 : Outport  Tag=outport/VisuCasingLights  Port=2  SampleTime=10/1000
  wires:
  VISUCasingLights_1_Mux/1(VISUCasingLights_1_TrafficLightDoubleUS_4) -> VISUCasingLights_1_TrafficLightDoubleUS_4/1
  VISUCasingLights_2_Mux/1(VISUCasingLights_2_TrafficLightDoubleUS_4) -> VISUCasingLights_2_TrafficLightDoubleUS_4/1
  Ground_1/1 -> VISUCasingLights_1_Mux/1(Green [-])
  Ground_2/1 -> VISUCasingLights_1_Mux/2(Orange [-])
  Ground_3/1 -> VISUCasingLights_1_Mux/3(Red [-])
  Ground_4/1 -> VISUCasingLights_2_Mux/1(Green [-])
  Ground_5/1 -> VISUCasingLights_2_Mux/2(Orange [-])
  Ground_6/1 -> VISUCasingLights_2_Mux/3(Red [-])

== system Straight_cs_old/VISUCasingLights_1_TrafficLightDoubleUS_1 ==
  VISUCasingLights_1_TrafficLightDoubleUS_1 : Inport  Tag=inport/VisuCasingLights  SampleTime=10/1000  BusOutputAsStruct=on
  Actuator : Subsystem  mask(PreScan Sink Block: VisuTrafficLight){UniqueID=1495, ColorsObjectQuery=, Colors=[]}
      mask prompts: UniqueID "Parent Unique Identifier"; ColorsObjectQuery "Query for Color Object"; Colors "Matrix of colors"
      mask help:
      | The VisuTrafficLight block provides a way to animate traffic lights: switch on and off individual lights.
      |
      | For more information, please click Help.
      mask Help: eval('openHelp(731)')
      mask Display: image(imread('TrafficLightCasing.png'))
  wires:
  VISUCasingLights_1_TrafficLightDoubleUS_1/1 -> Actuator/1(VISUCasingLights_1_TrafficLightDoubleUS_1)

== system Straight_cs_old/VISUCasingLights_1_TrafficLightDoubleUS_2 ==
  VISUCasingLights_1_TrafficLightDoubleUS_2 : Inport  Tag=inport/VisuCasingLights  SampleTime=10/1000  BusOutputAsStruct=on
  Actuator : Subsystem  mask(PreScan Sink Block: VisuTrafficLight){UniqueID=1496, ColorsObjectQuery=, Colors=[]}
      mask prompts: UniqueID "Parent Unique Identifier"; ColorsObjectQuery "Query for Color Object"; Colors "Matrix of colors"
      mask help:
      | The VisuTrafficLight block provides a way to animate traffic lights: switch on and off individual lights.
      |
      | For more information, please click Help.
      mask Help: eval('openHelp(731)')
      mask Display: image(imread('TrafficLightCasing.png'))
  wires:
  VISUCasingLights_1_TrafficLightDoubleUS_2/1 -> Actuator/1(VISUCasingLights_1_TrafficLightDoubleUS_2)

== system Straight_cs_old/VISUCasingLights_1_TrafficLightDoubleUS_3 ==
  VISUCasingLights_1_TrafficLightDoubleUS_3 : Inport  Tag=inport/VisuCasingLights  SampleTime=10/1000  BusOutputAsStruct=on
  Actuator : Subsystem  mask(PreScan Sink Block: VisuTrafficLight){UniqueID=1497, ColorsObjectQuery=, Colors=[]}
      mask prompts: UniqueID "Parent Unique Identifier"; ColorsObjectQuery "Query for Color Object"; Colors "Matrix of colors"
      mask help:
      | The VisuTrafficLight block provides a way to animate traffic lights: switch on and off individual lights.
      |
      | For more information, please click Help.
      mask Help: eval('openHelp(731)')
      mask Display: image(imread('TrafficLightCasing.png'))
  wires:
  VISUCasingLights_1_TrafficLightDoubleUS_3/1 -> Actuator/1(VISUCasingLights_1_TrafficLightDoubleUS_3)

== system Straight_cs_old/VISUCasingLights_1_TrafficLightDoubleUS_4 ==
  VISUCasingLights_1_TrafficLightDoubleUS_4 : Inport  Tag=inport/VisuCasingLights  SampleTime=10/1000  BusOutputAsStruct=on
  Actuator : Subsystem  mask(PreScan Sink Block: VisuTrafficLight){UniqueID=1498, ColorsObjectQuery=, Colors=[]}
      mask prompts: UniqueID "Parent Unique Identifier"; ColorsObjectQuery "Query for Color Object"; Colors "Matrix of colors"
      mask help:
      | The VisuTrafficLight block provides a way to animate traffic lights: switch on and off individual lights.
      |
      | For more information, please click Help.
      mask Help: eval('openHelp(731)')
      mask Display: image(imread('TrafficLightCasing.png'))
  wires:
  VISUCasingLights_1_TrafficLightDoubleUS_4/1 -> Actuator/1(VISUCasingLights_1_TrafficLightDoubleUS_4)

== system Straight_cs_old/VISUCasingLights_2_TrafficLightDoubleUS_1 ==
  VISUCasingLights_2_TrafficLightDoubleUS_1 : Inport  Tag=inport/VisuCasingLights  SampleTime=10/1000  BusOutputAsStruct=on
  Actuator : Subsystem  mask(PreScan Sink Block: VisuTrafficLight){UniqueID=1495, ColorsObjectQuery=, Colors=[]}
      mask prompts: UniqueID "Parent Unique Identifier"; ColorsObjectQuery "Query for Color Object"; Colors "Matrix of colors"
      mask help:
      | The VisuTrafficLight block provides a way to animate traffic lights: switch on and off individual lights.
      |
      | For more information, please click Help.
      mask Help: eval('openHelp(731)')
      mask Display: image(imread('TrafficLightCasing.png'))
  wires:
  VISUCasingLights_2_TrafficLightDoubleUS_1/1 -> Actuator/1(VISUCasingLights_2_TrafficLightDoubleUS_1)

== system Straight_cs_old/VISUCasingLights_2_TrafficLightDoubleUS_2 ==
  VISUCasingLights_2_TrafficLightDoubleUS_2 : Inport  Tag=inport/VisuCasingLights  SampleTime=10/1000  BusOutputAsStruct=on
  Actuator : Subsystem  mask(PreScan Sink Block: VisuTrafficLight){UniqueID=1496, ColorsObjectQuery=, Colors=[]}
      mask prompts: UniqueID "Parent Unique Identifier"; ColorsObjectQuery "Query for Color Object"; Colors "Matrix of colors"
      mask help:
      | The VisuTrafficLight block provides a way to animate traffic lights: switch on and off individual lights.
      |
      | For more information, please click Help.
      mask Help: eval('openHelp(731)')
      mask Display: image(imread('TrafficLightCasing.png'))
  wires:
  VISUCasingLights_2_TrafficLightDoubleUS_2/1 -> Actuator/1(VISUCasingLights_2_TrafficLightDoubleUS_2)

== system Straight_cs_old/VISUCasingLights_2_TrafficLightDoubleUS_3 ==
  VISUCasingLights_2_TrafficLightDoubleUS_3 : Inport  Tag=inport/VisuCasingLights  SampleTime=10/1000  BusOutputAsStruct=on
  Actuator : Subsystem  mask(PreScan Sink Block: VisuTrafficLight){UniqueID=1497, ColorsObjectQuery=, Colors=[]}
      mask prompts: UniqueID "Parent Unique Identifier"; ColorsObjectQuery "Query for Color Object"; Colors "Matrix of colors"
      mask help:
      | The VisuTrafficLight block provides a way to animate traffic lights: switch on and off individual lights.
      |
      | For more information, please click Help.
      mask Help: eval('openHelp(731)')
      mask Display: image(imread('TrafficLightCasing.png'))
  wires:
  VISUCasingLights_2_TrafficLightDoubleUS_3/1 -> Actuator/1(VISUCasingLights_2_TrafficLightDoubleUS_3)

== system Straight_cs_old/VISUCasingLights_2_TrafficLightDoubleUS_4 ==
  VISUCasingLights_2_TrafficLightDoubleUS_4 : Inport  Tag=inport/VisuCasingLights  SampleTime=10/1000  BusOutputAsStruct=on
  Actuator : Subsystem  mask(PreScan Sink Block: VisuTrafficLight){UniqueID=1498, ColorsObjectQuery=, Colors=[]}
      mask prompts: UniqueID "Parent Unique Identifier"; ColorsObjectQuery "Query for Color Object"; Colors "Matrix of colors"
      mask help:
      | The VisuTrafficLight block provides a way to animate traffic lights: switch on and off individual lights.
      |
      | For more information, please click Help.
      mask Help: eval('openHelp(731)')
      mask Display: image(imread('TrafficLightCasing.png'))
  wires:
  VISUCasingLights_2_TrafficLightDoubleUS_4/1 -> Actuator/1(VISUCasingLights_2_TrafficLightDoubleUS_4)

== system Straight_cs_old/WheelL0_Roewe_550_S_Sedan_1 ==
  WheelL0_Roewe_550_S_Sedan_1 : Inport  Tag=inport/JointActuator  OutDataTypeStr=Bus: PRESCAN_POSE_DATA  SampleTime=10/1000  BusOutputAsStruct=on
  Actuator : Subsystem  Tag=VisuJoint  mask(PreScan Sink Block: VisuJoint){UniqueID=29, Translate_ObjectID3D=Roewe_550_S_Sedan_1.WheelL0, Rotate_ObjectID3D=Roewe_550_S_Sedan_1.WheelL0, TimeStep=10/1000, DisplayName=[]}
      mask prompts: UniqueID "Parent Unique ID"; Translate_ObjectID3D "Translate Object Name"; Rotate_ObjectID3D "Rotate Object Name"; TimeStep "Simulation Step"; DisplayName "Display Name"
      mask help:
      | The VisuJoint block provides a way to adapt the location and orientation of a part of an object.
      |
      | For more information, please click Help.
      settings: DeleteFcn=PreScanBlockDeleteFcn;
      mask Help: eval('openHelp(223)')
      mask Display: image(imread('Joint.png'))
  wires:
  WheelL0_Roewe_550_S_Sedan_1/1 -> Actuator/1(Joint)

== system Straight_cs_old/WheelL1_Roewe_550_S_Sedan_1 ==
  WheelL1_Roewe_550_S_Sedan_1 : Inport  Tag=inport/JointActuator  OutDataTypeStr=Bus: PRESCAN_POSE_DATA  SampleTime=10/1000  BusOutputAsStruct=on
  Actuator : Subsystem  Tag=VisuJoint  mask(PreScan Sink Block: VisuJoint){UniqueID=29, Translate_ObjectID3D=Roewe_550_S_Sedan_1.WheelL1, Rotate_ObjectID3D=Roewe_550_S_Sedan_1.WheelL1, TimeStep=10/1000, DisplayName=[]}
      mask prompts: UniqueID "Parent Unique ID"; Translate_ObjectID3D "Translate Object Name"; Rotate_ObjectID3D "Rotate Object Name"; TimeStep "Simulation Step"; DisplayName "Display Name"
      mask help:
      | The VisuJoint block provides a way to adapt the location and orientation of a part of an object.
      |
      | For more information, please click Help.
      settings: DeleteFcn=PreScanBlockDeleteFcn;
      mask Help: eval('openHelp(223)')
      mask Display: image(imread('Joint.png'))
  wires:
  WheelL1_Roewe_550_S_Sedan_1/1 -> Actuator/1(Joint)

== system Straight_cs_old/WheelR0_Roewe_550_S_Sedan_1 ==
  WheelR0_Roewe_550_S_Sedan_1 : Inport  Tag=inport/JointActuator  OutDataTypeStr=Bus: PRESCAN_POSE_DATA  SampleTime=10/1000  BusOutputAsStruct=on
  Actuator : Subsystem  Tag=VisuJoint  mask(PreScan Sink Block: VisuJoint){UniqueID=29, Translate_ObjectID3D=Roewe_550_S_Sedan_1.WheelR0, Rotate_ObjectID3D=Roewe_550_S_Sedan_1.WheelR0, TimeStep=10/1000, DisplayName=[]}
      mask prompts: UniqueID "Parent Unique ID"; Translate_ObjectID3D "Translate Object Name"; Rotate_ObjectID3D "Rotate Object Name"; TimeStep "Simulation Step"; DisplayName "Display Name"
      mask help:
      | The VisuJoint block provides a way to adapt the location and orientation of a part of an object.
      |
      | For more information, please click Help.
      settings: DeleteFcn=PreScanBlockDeleteFcn;
      mask Help: eval('openHelp(223)')
      mask Display: image(imread('Joint.png'))
  wires:
  WheelR0_Roewe_550_S_Sedan_1/1 -> Actuator/1(Joint)

== system Straight_cs_old/WheelR1_Roewe_550_S_Sedan_1 ==
  WheelR1_Roewe_550_S_Sedan_1 : Inport  Tag=inport/JointActuator  OutDataTypeStr=Bus: PRESCAN_POSE_DATA  SampleTime=10/1000  BusOutputAsStruct=on
  Actuator : Subsystem  Tag=VisuJoint  mask(PreScan Sink Block: VisuJoint){UniqueID=29, Translate_ObjectID3D=Roewe_550_S_Sedan_1.WheelR1, Rotate_ObjectID3D=Roewe_550_S_Sedan_1.WheelR1, TimeStep=10/1000, DisplayName=[]}
      mask prompts: UniqueID "Parent Unique ID"; Translate_ObjectID3D "Translate Object Name"; Rotate_ObjectID3D "Rotate Object Name"; TimeStep "Simulation Step"; DisplayName "Display Name"
      mask help:
      | The VisuJoint block provides a way to adapt the location and orientation of a part of an object.
      |
      | For more information, please click Help.
      settings: DeleteFcn=PreScanBlockDeleteFcn;
      mask Help: eval('openHelp(223)')
      mask Display: image(imread('Joint.png'))
  wires:
  WheelR1_Roewe_550_S_Sedan_1/1 -> Actuator/1(Joint)

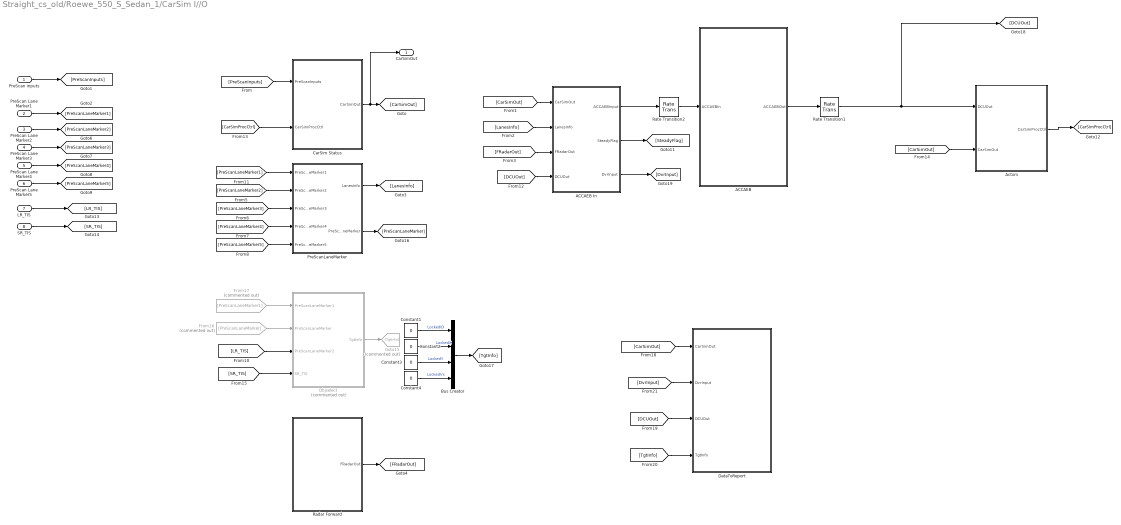
== system Straight_cs_old/Roewe_550_S_Sedan_1/CarSim I//O ==
  PreScan inputs : Inport
  PreScan Lane Marker1 : Inport  Port=2
  PreScan Lane Marker2 : Inport  Port=3
  PreScan Lane Marker3 : Inport  Port=4
  PreScan Lane Marker4 : Inport  Port=5
  PreScan Lane Marker5 : Inport  Port=6
  LR_TIS : Inport  Port=7
  SR_TIS : Inport  Port=8
  ACCAEB : Subsystem  DialogController=pil_create_dialog  LoadFcn=|
      | try
      |    if ~strcmp(rtw.pil.getPILVersion, '6.10 (R2016a)_12')
      |       set_param(gcb, 'DialogController', '');
      |       set_param(gcb, 'DialogControllerArgs', '');
      |    end
      | catch e
      |       set_param(gcb, 'DialogController', '');
      |       set_param(gcb, 'DialogControllerArgs', '');
      | end
      mask help: PIL:pil:XILBlockMaskDesc
      mask Display: disp('SIL S-Function');
  ACCAEB In : Subsystem  TreatAsAtomicUnit=on
  Actors : Subsystem
  Bus Creator : BusCreator  Inputs=4
  "CarSim Status " : Subsystem  TreatAsAtomicUnit=on
  Constant{1..4} (4 alike) : Constant  Value=0
  DataToReport : Subsystem  TreatAsAtomicUnit=on  SystemSampleTime=0.05
  From16 : From  Commented=on  GotoTag=PreScanLaneMarker
  From17 : From  Commented=on  GotoTag=PreScanLaneMarker1
  Goto15 : Goto  Commented=on  GotoTag=TgtInfo
  Objselect : Subsystem  Commented=on
  PreScanLaneMarker : Subsystem  TreatAsAtomicUnit=on
  Radar Forward : Subsystem  TreatAsAtomicUnit=on
  Rate Transition1 : RateTransition  OutPortSampleTime=0.001
  Rate Transition2 : RateTransition  OutPortSampleTime=0.01
  CarSimOut : Outport
  wires:
  [PreScanInputs] -> "CarSim Status "/1(PreScanInputs)
  PreScan inputs/1 -> [PreScanInputs]
  PreScan Lane Marker1/1 -> [PreScanLaneMarker1]
  "CarSim Status "/1(CarSimOut) -> CarSimOut/1, [CarSimOut]
  [PreScanLaneMarker1] -> PreScanLaneMarker/1(PreScanLaneMarker1)
  [CarSimOut] -> ACCAEB In/1(CarSimOut)
  PreScanLaneMarker/1(LanesInfo) -> [LanesInfo]
  [LanesInfo] -> ACCAEB In/2(LanesInfo)
  Radar Forward/1(FRadarOut) -> [FRadarOut]
  [FRadarOut] -> ACCAEB In/3(FRadarOut)
  [CarSimProcCtrl] -> "CarSim Status "/2(CarSimProcCtrl)
  PreScan Lane Marker2/1 -> [PreScanLaneMarker2]
  PreScan Lane Marker3/1 -> [PreScanLaneMarker3]
  PreScan Lane Marker4/1 -> [PreScanLaneMarker4]
  PreScan Lane Marker5/1 -> [PreScanLaneMarker5]
  [PreScanLaneMarker2] -> PreScanLaneMarker/2(PreScanLaneMarker2)
  [PreScanLaneMarker3] -> PreScanLaneMarker/3(PreScanLaneMarker3)
  [PreScanLaneMarker4] -> PreScanLaneMarker/4(PreScanLaneMarker4)
  [PreScanLaneMarker5] -> PreScanLaneMarker/5(PreScanLaneMarker5)
  Rate Transition2/1 -> ACCAEB/1(ACCAEBIn)
  ACCAEB In/1(ACCAEBInput) -> Rate Transition2/1
  ACCAEB/1(ACCAEBOut) -> Rate Transition1/1
  ACCAEB In/2(SteadyFlag) -> [SteadyFlag]
  [CarSimOut] -> Actors/2(CarSimOut)
  Actors/1(CarSimProcCtrl) -> [CarSimProcCtrl]
  [DCUOut] -> ACCAEB In/4(DCUOut)
  LR_TIS/1 -> [LR_TIS]
  SR_TIS/1 -> [SR_TIS]
  From16/1 -> Objselect/2(PreScanLaneMarker)
  From17/1 -> Objselect/1(PreScanLaneMarker1)
  Objselect/1(TgtInfo) -> Goto15/1
  [LR_TIS] -> Objselect/3(PreScanLaneMarker2)
  [SR_TIS] -> Objselect/4(SR_TIS)
  PreScanLaneMarker/2(PreScanLaneMarker) -> [PreScanLaneMarker]
  Bus Creator/1 -> [TgtInfo]
  Constant1/1 -> Bus Creator/1  "LockedID"
  Constant2/1 -> Bus Creator/2  "LockedX"
  Constant3/1 -> Bus Creator/3  "LockedY"
  Constant4/1 -> Bus Creator/4  "LockedVx"
  [DvrInput] -> DataToReport/2(DvrInput)
  [CarSimOut] -> DataToReport/1(CarSimOut)
  [DCUOut] -> DataToReport/3(DCUOut)
  [TgtInfo] -> DataToReport/4(TgtInfo)
  Rate Transition1/1 -> [DCUOut], Actors/1(DCUOut)
  ACCAEB In/3(DvrInput) -> [DvrInput]
